simulink model "Charge_1_V1_experiment"  (R2018b)
settings: Solver=FixedStepDiscrete  StartTime=0.0  StopTime=1  FixedStep=0.001  RelTol=1e-3
PreLoadFcn:
  | librarySetup
  | eval([bdroot,'_startup']) %Calling [modelName]_startup.m
undefined symbols (not defined in the file or in its folder): A0, A1, Car1__Authorize, Car2_Authorize, CON2, CON3, CON4, Control_Mode_In, CurrentSP, D10, D12, D13, D2, D3, D4, D5, D6, D7, D8, Free_Charge, Frequency_High_Point, Frequency_Low_Point, Frequency_Mid_high, Frequency_Mid_low, HVol_High_Point, HVol_Low_Point, HVol_Mid_high, HVol_Mid_low, HVoltage_Factor, SeconCar_ThreePhase, V_Current_five, V_Current_four, V_Current_one, V_Current_six, V_Current_three, V_Current_two, V_Frequency, V_MaxPliot, V_MinPliot, Vol_High_Point, Vol_Low_Point, Vol_Mid_high, Vol_Mid_low, Voltage_Factor, Voltage_Mode_Test
libraries: simulink x324, HANcoder_STM32_Target x30, powerlib_meascontrol x8, simulink_extras x2
(part 10 of 13)

== system Charge_1_V1_experiment/HANcoder STM32 Target - E407-STM32 algorithm/Energy Meter/Energy_Meter_Recieve/Subsystem1/f1/Last byte ==
  note: 01040000000271CB
  Trigger : TriggerPort  VariantControl=Variant
  Constant1 : Constant  Value=hex2dec('0A')  OutDataTypeStr=uint8  SampleTime=-1
  UART send : Subsystem  Tag=HANcoder_TARGET_STM32_E407  AncestorBlock=HANcoder_STM32_Target/STM32-E407/UART/UART send  mask(UART send){channel=UART1: CON3 - D1 & D0, useStatusOut=off, tsamp=-1}
      mask prompts: useStatusOut "Use status outport"; tsamp "Sample time"
      mask help:
      | Function
      | ==========
      | Transmits a byte on the UART communication interface.
      |
      | Parameters per channel
      | ======================
      | - Select channel (TX & RX)
      | - Select if the status output should be enabled.
      |
      | Inputs
      | ======
      | - The byte to send
      |
      | Outputs
      | =======
      | - When the status output is 0, the byte could not be transmitted. Probably
      |   because the transmit buffer was configured too small.
      mask init:
      | uartChannelInfoStr = sfcn_uart_send_mcb(2, channel, useStatusOut);
      settings: MoveFcn=drawLogos
      mask Help: web('sfcn_uart_send.html')
      mask TypeOptions channel: UART1: CON3 - D1 & D0 | UART2: CON PD - 8 & 9 | UART3: CON PD - 11 & 12 | UART6: UEXT - 3 & 4
      mask Display: fprintf('UART send\n%s', uartChannelInfoStr);patch([245 251 251],[8 14 2],[1 0 0]);patch([253 253 259],[14 2 8],[0 0 0.35]);
  wires:
  Constant1/1 -> UART send/1(In1)

== system Charge_1_V1_experiment/HANcoder STM32 Target - E407-STM32 algorithm/Energy Meter/Energy_Meter_Recieve/Subsystem1/f1/Read_Gyro11 ==
  Trigger : TriggerPort  VariantControl=Variant
  Constant : Constant  Value=hex2dec('0E')  OutDataTypeStr=uint8  SampleTime=-1
  UART send : Subsystem  Tag=HANcoder_TARGET_STM32_E407  AncestorBlock=HANcoder_STM32_Target/STM32-E407/UART/UART send  mask(UART send){channel=UART1: CON3 - D1 & D0, useStatusOut=off, tsamp=-1}
      mask prompts: useStatusOut "Use status outport"; tsamp "Sample time"
      mask help:
      | Function
      | ==========
      | Transmits a byte on the UART communication interface.
      |
      | Parameters per channel
      | ======================
      | - Select channel (TX & RX)
      | - Select if the status output should be enabled.
      |
      | Inputs
      | ======
      | - The byte to send
      |
      | Outputs
      | =======
      | - When the status output is 0, the byte could not be transmitted. Probably
      |   because the transmit buffer was configured too small.
      mask init:
      | uartChannelInfoStr = sfcn_uart_send_mcb(2, channel, useStatusOut);
      settings: MoveFcn=drawLogos
      mask Help: web('sfcn_uart_send.html')
      mask TypeOptions channel: UART1: CON3 - D1 & D0 | UART2: CON PD - 8 & 9 | UART3: CON PD - 11 & 12 | UART6: UEXT - 3 & 4
      mask Display: fprintf('UART send\n%s', uartChannelInfoStr);patch([245 251 251],[8 14 2],[1 0 0]);patch([253 253 259],[14 2 8],[0 0 0.35]);
  wires:
  Constant/1 -> UART send/1(In1)

== system Charge_1_V1_experiment/HANcoder STM32 Target - E407-STM32 algorithm/Energy Meter/Energy_Meter_Recieve/Subsystem1/f1/Read_Gyro6 ==
  Trigger : TriggerPort  VariantControl=Variant
  Constant : Constant  Value=hex2dec('2')  OutDataTypeStr=uint8  SampleTime=-1
  UART send : Subsystem  Tag=HANcoder_TARGET_STM32_E407  AncestorBlock=HANcoder_STM32_Target/STM32-E407/UART/UART send  mask(UART send){channel=UART1: CON3 - D1 & D0, useStatusOut=off, tsamp=-1}
      mask prompts: useStatusOut "Use status outport"; tsamp "Sample time"
      mask help:
      | Function
      | ==========
      | Transmits a byte on the UART communication interface.
      |
      | Parameters per channel
      | ======================
      | - Select channel (TX & RX)
      | - Select if the status output should be enabled.
      |
      | Inputs
      | ======
      | - The byte to send
      |
      | Outputs
      | =======
      | - When the status output is 0, the byte could not be transmitted. Probably
      |   because the transmit buffer was configured too small.
      mask init:
      | uartChannelInfoStr = sfcn_uart_send_mcb(2, channel, useStatusOut);
      settings: MoveFcn=drawLogos
      mask Help: web('sfcn_uart_send.html')
      mask TypeOptions channel: UART1: CON3 - D1 & D0 | UART2: CON PD - 8 & 9 | UART3: CON PD - 11 & 12 | UART6: UEXT - 3 & 4
      mask Display: fprintf('UART send\n%s', uartChannelInfoStr);patch([245 251 251],[8 14 2],[1 0 0]);patch([253 253 259],[14 2 8],[0 0 0.35]);
  wires:
  Constant/1 -> UART send/1(In1)

== system Charge_1_V1_experiment/HANcoder STM32 Target - E407-STM32 algorithm/Energy Meter/Energy_Meter_Recieve/Subsystem1/f1/Subsystem ==
  In1 : Inport
  In10 : Inport  Port=2
  In11 : Inport  Port=3
  In12 : Inport  Port=4
  In13 : Inport  Port=5
  Compare To Constant10 : simulink/Logic and Bit Operations/Compare To Constant  relop===  const=411  OutDataTypeStr=boolean
  Compare To Constant11 : simulink/Logic and Bit Operations/Compare To Constant  relop===  const=412  OutDataTypeStr=boolean
  Compare To Constant13 : simulink/Logic and Bit Operations/Compare To Constant  relop===  const=413  OutDataTypeStr=boolean
  Compare To Constant9 : simulink/Logic and Bit Operations/Compare To Constant  relop===  const=410  OutDataTypeStr=boolean
  Read_Gyro10 : Subsystem  TreatAsAtomicUnit=on
  Read_Gyro12 : Subsystem  TreatAsAtomicUnit=on
  Read_Gyro13 : Subsystem  TreatAsAtomicUnit=on
  Read_Gyro14 : Subsystem  TreatAsAtomicUnit=on
  wires:
  In13/1 -> Read_Gyro14/1(In1)
  Compare To Constant13/1 -> Read_Gyro14/Trigger
  Compare To Constant11/1 -> Read_Gyro13/Trigger
  Compare To Constant9/1 -> Read_Gyro10/Trigger
  Compare To Constant10/1 -> Read_Gyro12/Trigger
  In12/1 -> Read_Gyro13/1(In1)
  In11/1 -> Read_Gyro12/1(In1)
  In10/1 -> Read_Gyro10/1(In1)
  In1/1 -> Compare To Constant9/1, Compare To Constant10/1, Compare To Constant11/1, Compare To Constant13/1

== system Charge_1_V1_experiment/HANcoder STM32 Target - E407-STM32 algorithm/Energy Meter/Energy_Meter_Recieve/Subsystem1/f2/Current_Phase1 ==
  In1 : Inport
  In2 : Inport  Port=2
  In3 : Inport  Port=3
  In4 : Inport  Port=4
  In5 : Inport  Port=5
  Compare To Constant1 : simulink/Logic and Bit Operations/Compare To Constant  relop===  const=603  OutDataTypeStr=boolean
  Compare To Constant12 : simulink/Logic and Bit Operations/Compare To Constant  relop===  const=602  OutDataTypeStr=boolean
  Compare To Constant2 : simulink/Logic and Bit Operations/Compare To Constant  relop===  const=604  OutDataTypeStr=boolean
  Compare To Constant3 : simulink/Logic and Bit Operations/Compare To Constant  relop===  const=605  OutDataTypeStr=boolean
  Read_Gyro1 : Subsystem  TreatAsAtomicUnit=on
  Read_Gyro2 : Subsystem  TreatAsAtomicUnit=on
  Read_Gyro3 : Subsystem  TreatAsAtomicUnit=on
  Read_Gyro4 : Subsystem  TreatAsAtomicUnit=on
  wires:
  In3/1 -> Read_Gyro2/1(In1)
  In2/1 -> Read_Gyro1/1(In1)
  Compare To Constant1/1 -> Read_Gyro2/Trigger
  Compare To Constant3/1 -> Read_Gyro4/Trigger
  Compare To Constant2/1 -> Read_Gyro3/Trigger
  In5/1 -> Read_Gyro4/1(In1)
  In4/1 -> Read_Gyro3/1(In1)
  Compare To Constant12/1 -> Read_Gyro1/Trigger
  In1/1 -> Compare To Constant3/1, Compare To Constant2/1, Compare To Constant1/1, Compare To Constant12/1

== system Charge_1_V1_experiment/HANcoder STM32 Target - E407-STM32 algorithm/Energy Meter/Energy_Meter_Recieve/Subsystem1/f2/Last byte ==
  note: 01040000000271CB
  Trigger : TriggerPort  VariantControl=Variant
  Constant1 : Constant  Value=hex2dec('0A')  OutDataTypeStr=uint8  SampleTime=-1
  UART send : Subsystem  Tag=HANcoder_TARGET_STM32_E407  AncestorBlock=HANcoder_STM32_Target/STM32-E407/UART/UART send  mask(UART send){channel=UART1: CON3 - D1 & D0, useStatusOut=off, tsamp=-1}
      mask prompts: useStatusOut "Use status outport"; tsamp "Sample time"
      mask help:
      | Function
      | ==========
      | Transmits a byte on the UART communication interface.
      |
      | Parameters per channel
      | ======================
      | - Select channel (TX & RX)
      | - Select if the status output should be enabled.
      |
      | Inputs
      | ======
      | - The byte to send
      |
      | Outputs
      | =======
      | - When the status output is 0, the byte could not be transmitted. Probably
      |   because the transmit buffer was configured too small.
      mask init:
      | uartChannelInfoStr = sfcn_uart_send_mcb(2, channel, useStatusOut);
      settings: MoveFcn=drawLogos
      mask Help: web('sfcn_uart_send.html')
      mask TypeOptions channel: UART1: CON3 - D1 & D0 | UART2: CON PD - 8 & 9 | UART3: CON PD - 11 & 12 | UART6: UEXT - 3 & 4
      mask Display: fprintf('UART send\n%s', uartChannelInfoStr);patch([245 251 251],[8 14 2],[1 0 0]);patch([253 253 259],[14 2 8],[0 0 0.35]);
  wires:
  Constant1/1 -> UART send/1(In1)

== system Charge_1_V1_experiment/HANcoder STM32 Target - E407-STM32 algorithm/Energy Meter/Energy_Meter_Recieve/Subsystem1/f2/Read_Gyro11 ==
  Trigger : TriggerPort  VariantControl=Variant
  Constant : Constant  Value=hex2dec('0F')  OutDataTypeStr=uint8  SampleTime=-1
  UART send : Subsystem  Tag=HANcoder_TARGET_STM32_E407  AncestorBlock=HANcoder_STM32_Target/STM32-E407/UART/UART send  mask(UART send){channel=UART1: CON3 - D1 & D0, useStatusOut=off, tsamp=-1}
      mask prompts: useStatusOut "Use status outport"; tsamp "Sample time"
      mask help:
      | Function
      | ==========
      | Transmits a byte on the UART communication interface.
      |
      | Parameters per channel
      | ======================
      | - Select channel (TX & RX)
      | - Select if the status output should be enabled.
      |
      | Inputs
      | ======
      | - The byte to send
      |
      | Outputs
      | =======
      | - When the status output is 0, the byte could not be transmitted. Probably
      |   because the transmit buffer was configured too small.
      mask init:
      | uartChannelInfoStr = sfcn_uart_send_mcb(2, channel, useStatusOut);
      settings: MoveFcn=drawLogos
      mask Help: web('sfcn_uart_send.html')
      mask TypeOptions channel: UART1: CON3 - D1 & D0 | UART2: CON PD - 8 & 9 | UART3: CON PD - 11 & 12 | UART6: UEXT - 3 & 4
      mask Display: fprintf('UART send\n%s', uartChannelInfoStr);patch([245 251 251],[8 14 2],[1 0 0]);patch([253 253 259],[14 2 8],[0 0 0.35]);
  wires:
  Constant/1 -> UART send/1(In1)

== system Charge_1_V1_experiment/HANcoder STM32 Target - E407-STM32 algorithm/Energy Meter/Energy_Meter_Recieve/Subsystem1/f2/Read_Gyro6 ==
  Trigger : TriggerPort  VariantControl=Variant
  Constant : Constant  Value=hex2dec('3')  OutDataTypeStr=uint8  SampleTime=-1
  UART send : Subsystem  Tag=HANcoder_TARGET_STM32_E407  AncestorBlock=HANcoder_STM32_Target/STM32-E407/UART/UART send  mask(UART send){channel=UART1: CON3 - D1 & D0, useStatusOut=off, tsamp=-1}
      mask prompts: useStatusOut "Use status outport"; tsamp "Sample time"
      mask help:
      | Function
      | ==========
      | Transmits a byte on the UART communication interface.
      |
      | Parameters per channel
      | ======================
      | - Select channel (TX & RX)
      | - Select if the status output should be enabled.
      |
      | Inputs
      | ======
      | - The byte to send
      |
      | Outputs
      | =======
      | - When the status output is 0, the byte could not be transmitted. Probably
      |   because the transmit buffer was configured too small.
      mask init:
      | uartChannelInfoStr = sfcn_uart_send_mcb(2, channel, useStatusOut);
      settings: MoveFcn=drawLogos
      mask Help: web('sfcn_uart_send.html')
      mask TypeOptions channel: UART1: CON3 - D1 & D0 | UART2: CON PD - 8 & 9 | UART3: CON PD - 11 & 12 | UART6: UEXT - 3 & 4
      mask Display: fprintf('UART send\n%s', uartChannelInfoStr);patch([245 251 251],[8 14 2],[1 0 0]);patch([253 253 259],[14 2 8],[0 0 0.35]);
  wires:
  Constant/1 -> UART send/1(In1)

== system Charge_1_V1_experiment/HANcoder STM32 Target - E407-STM32 algorithm/Energy Meter/Energy_Meter_Recieve/Voltage_meter1/Read_Gyro/UART receive ==
  Level-2 M-file S-Function : M-S-Function  Tag=XECU_TARGET_STM32_E407  FunctionName=sfcn_uart_receive  Parameters=tsamp
  Term1 : Terminator
  Out1 : Outport
  wires:
  Level-2 M-file S-Function/2 -> Term1/1
  Level-2 M-file S-Function/1 -> Out1/1

== system Charge_1_V1_experiment/HANcoder STM32 Target - E407-STM32 algorithm/Energy Meter/Energy_Meter_Recieve/Voltage_meter1/Read_Gyro1/UART receive ==
  Level-2 M-file S-Function : M-S-Function  Tag=XECU_TARGET_STM32_E407  FunctionName=sfcn_uart_receive  Parameters=tsamp
  Term1 : Terminator
  Out1 : Outport
  wires:
  Level-2 M-file S-Function/2 -> Term1/1
  Level-2 M-file S-Function/1 -> Out1/1

== system Charge_1_V1_experiment/HANcoder STM32 Target - E407-STM32 algorithm/Energy Meter/Energy_Meter_Recieve/Voltage_meter1/Read_Gyro10/UART receive ==
  Level-2 M-file S-Function : M-S-Function  Tag=XECU_TARGET_STM32_E407  FunctionName=sfcn_uart_receive  Parameters=tsamp
  Term1 : Terminator
  Out1 : Outport
  wires:
  Level-2 M-file S-Function/2 -> Term1/1
  Level-2 M-file S-Function/1 -> Out1/1

== system Charge_1_V1_experiment/HANcoder STM32 Target - E407-STM32 algorithm/Energy Meter/Energy_Meter_Recieve/Voltage_meter1/Read_Gyro11/UART receive ==
  Level-2 M-file S-Function : M-S-Function  Tag=XECU_TARGET_STM32_E407  FunctionName=sfcn_uart_receive  Parameters=tsamp
  Term1 : Terminator
  Out1 : Outport
  wires:
  Level-2 M-file S-Function/1 -> Out1/1
  Level-2 M-file S-Function/2 -> Term1/1

== system Charge_1_V1_experiment/HANcoder STM32 Target - E407-STM32 algorithm/Energy Meter/Energy_Meter_Recieve/Voltage_meter1/Read_Gyro12/UART receive ==
  Level-2 M-file S-Function : M-S-Function  Tag=XECU_TARGET_STM32_E407  FunctionName=sfcn_uart_receive  Parameters=tsamp
  Term1 : Terminator
  Out1 : Outport
  wires:
  Level-2 M-file S-Function/2 -> Term1/1
  Level-2 M-file S-Function/1 -> Out1/1

== system Charge_1_V1_experiment/HANcoder STM32 Target - E407-STM32 algorithm/Energy Meter/Energy_Meter_Recieve/Voltage_meter1/Read_Gyro13/UART receive ==
  Level-2 M-file S-Function : M-S-Function  Tag=XECU_TARGET_STM32_E407  FunctionName=sfcn_uart_receive  Parameters=tsamp
  Term1 : Terminator
  Out1 : Outport
  wires:
  Level-2 M-file S-Function/1 -> Out1/1
  Level-2 M-file S-Function/2 -> Term1/1

== system Charge_1_V1_experiment/HANcoder STM32 Target - E407-STM32 algorithm/Energy Meter/Energy_Meter_Recieve/Voltage_meter1/Read_Gyro14/UART receive ==
  Level-2 M-file S-Function : M-S-Function  Tag=XECU_TARGET_STM32_E407  FunctionName=sfcn_uart_receive  Parameters=tsamp
  Term1 : Terminator
  Out1 : Outport
  wires:
  Level-2 M-file S-Function/2 -> Term1/1
  Level-2 M-file S-Function/1 -> Out1/1

== system Charge_1_V1_experiment/HANcoder STM32 Target - E407-STM32 algorithm/Energy Meter/Energy_Meter_Recieve/Voltage_meter1/Read_Gyro15/UART receive ==
  Level-2 M-file S-Function : M-S-Function  Tag=XECU_TARGET_STM32_E407  FunctionName=sfcn_uart_receive  Parameters=tsamp
  Term1 : Terminator
  Out1 : Outport
  wires:
  Level-2 M-file S-Function/1 -> Out1/1
  Level-2 M-file S-Function/2 -> Term1/1

== system Charge_1_V1_experiment/HANcoder STM32 Target - E407-STM32 algorithm/Energy Meter/Energy_Meter_Recieve/Voltage_meter1/Read_Gyro16/UART receive ==
  Level-2 M-file S-Function : M-S-Function  Tag=XECU_TARGET_STM32_E407  FunctionName=sfcn_uart_receive  Parameters=tsamp
  Term1 : Terminator
  Out1 : Outport
  wires:
  Level-2 M-file S-Function/2 -> Term1/1
  Level-2 M-file S-Function/1 -> Out1/1

== system Charge_1_V1_experiment/HANcoder STM32 Target - E407-STM32 algorithm/Energy Meter/Energy_Meter_Recieve/Voltage_meter1/Read_Gyro17/UART receive ==
  Level-2 M-file S-Function : M-S-Function  Tag=XECU_TARGET_STM32_E407  FunctionName=sfcn_uart_receive  Parameters=tsamp
  Term1 : Terminator
  Out1 : Outport
  wires:
  Level-2 M-file S-Function/1 -> Out1/1
  Level-2 M-file S-Function/2 -> Term1/1

== system Charge_1_V1_experiment/HANcoder STM32 Target - E407-STM32 algorithm/Energy Meter/Energy_Meter_Recieve/Voltage_meter1/Read_Gyro2/UART receive ==
  Level-2 M-file S-Function : M-S-Function  Tag=XECU_TARGET_STM32_E407  FunctionName=sfcn_uart_receive  Parameters=tsamp
  Term1 : Terminator
  Out1 : Outport
  wires:
  Level-2 M-file S-Function/2 -> Term1/1
  Level-2 M-file S-Function/1 -> Out1/1

== system Charge_1_V1_experiment/HANcoder STM32 Target - E407-STM32 algorithm/Energy Meter/Energy_Meter_Recieve/Voltage_meter1/Read_Gyro3/UART receive ==
  Level-2 M-file S-Function : M-S-Function  Tag=XECU_TARGET_STM32_E407  FunctionName=sfcn_uart_receive  Parameters=tsamp
  Term1 : Terminator
  Out1 : Outport
  wires:
  Level-2 M-file S-Function/2 -> Term1/1
  Level-2 M-file S-Function/1 -> Out1/1

== system Charge_1_V1_experiment/HANcoder STM32 Target - E407-STM32 algorithm/Energy Meter/Energy_Meter_Recieve/Voltage_meter1/Read_Gyro4/UART receive ==
  Level-2 M-file S-Function : M-S-Function  Tag=XECU_TARGET_STM32_E407  FunctionName=sfcn_uart_receive  Parameters=tsamp
  Term1 : Terminator
  Out1 : Outport
  wires:
  Level-2 M-file S-Function/2 -> Term1/1
  Level-2 M-file S-Function/1 -> Out1/1

== system Charge_1_V1_experiment/HANcoder STM32 Target - E407-STM32 algorithm/Energy Meter/Energy_Meter_Recieve/Voltage_meter1/Read_Gyro5/UART receive ==
  Level-2 M-file S-Function : M-S-Function  Tag=XECU_TARGET_STM32_E407  FunctionName=sfcn_uart_receive  Parameters=tsamp
  Term1 : Terminator
  Out1 : Outport
  wires:
  Level-2 M-file S-Function/2 -> Term1/1
  Level-2 M-file S-Function/1 -> Out1/1

== system Charge_1_V1_experiment/HANcoder STM32 Target - E407-STM32 algorithm/Energy Meter/Energy_Meter_Recieve/Voltage_meter1/Read_Gyro6/UART receive ==
  Level-2 M-file S-Function : M-S-Function  Tag=XECU_TARGET_STM32_E407  FunctionName=sfcn_uart_receive  Parameters=tsamp
  Term1 : Terminator
  Out1 : Outport
  wires:
  Level-2 M-file S-Function/2 -> Term1/1
  Level-2 M-file S-Function/1 -> Out1/1

== system Charge_1_V1_experiment/HANcoder STM32 Target - E407-STM32 algorithm/Energy Meter/Energy_Meter_Recieve/Voltage_meter1/Read_Gyro7/UART receive ==
  Level-2 M-file S-Function : M-S-Function  Tag=XECU_TARGET_STM32_E407  FunctionName=sfcn_uart_receive  Parameters=tsamp
  Term1 : Terminator
  Out1 : Outport
  wires:
  Level-2 M-file S-Function/2 -> Term1/1
  Level-2 M-file S-Function/1 -> Out1/1

== system Charge_1_V1_experiment/HANcoder STM32 Target - E407-STM32 algorithm/Energy Meter/Energy_Meter_Recieve/Voltage_meter1/Read_Gyro8/UART receive ==
  Level-2 M-file S-Function : M-S-Function  Tag=XECU_TARGET_STM32_E407  FunctionName=sfcn_uart_receive  Parameters=tsamp
  Term1 : Terminator
  Out1 : Outport
  wires:
  Level-2 M-file S-Function/2 -> Term1/1
  Level-2 M-file S-Function/1 -> Out1/1

== system Charge_1_V1_experiment/HANcoder STM32 Target - E407-STM32 algorithm/Energy Meter/Energy_Meter_Recieve/Voltage_meter1/Read_Gyro9/UART receive ==
  Level-2 M-file S-Function : M-S-Function  Tag=XECU_TARGET_STM32_E407  FunctionName=sfcn_uart_receive  Parameters=tsamp
  Term1 : Terminator
  Out1 : Outport
  wires:
  Level-2 M-file S-Function/2 -> Term1/1
  Level-2 M-file S-Function/1 -> Out1/1

== system Charge_1_V1_experiment/HANcoder STM32 Target - E407-STM32 algorithm/Energy Meter/Energy_Meter_Recieve/Voltage_meter2/Read_Gyro/UART receive ==
  Level-2 M-file S-Function : M-S-Function  Tag=XECU_TARGET_STM32_E407  FunctionName=sfcn_uart_receive  Parameters=tsamp
  Term1 : Terminator
  Out1 : Outport
  wires:
  Level-2 M-file S-Function/1 -> Out1/1
  Level-2 M-file S-Function/2 -> Term1/1

== system Charge_1_V1_experiment/HANcoder STM32 Target - E407-STM32 algorithm/Energy Meter/Energy_Meter_Recieve/Voltage_meter2/Read_Gyro1/UART receive ==
  Level-2 M-file S-Function : M-S-Function  Tag=XECU_TARGET_STM32_E407  FunctionName=sfcn_uart_receive  Parameters=tsamp
  Term1 : Terminator
  Out1 : Outport
  wires:
  Level-2 M-file S-Function/1 -> Out1/1
  Level-2 M-file S-Function/2 -> Term1/1

== system Charge_1_V1_experiment/HANcoder STM32 Target - E407-STM32 algorithm/Energy Meter/Energy_Meter_Recieve/Voltage_meter2/Read_Gyro10/UART receive ==
  Level-2 M-file S-Function : M-S-Function  Tag=XECU_TARGET_STM32_E407  FunctionName=sfcn_uart_receive  Parameters=tsamp
  Term1 : Terminator
  Out1 : Outport
  wires:
  Level-2 M-file S-Function/1 -> Out1/1
  Level-2 M-file S-Function/2 -> Term1/1

== system Charge_1_V1_experiment/HANcoder STM32 Target - E407-STM32 algorithm/Energy Meter/Energy_Meter_Recieve/Voltage_meter2/Read_Gyro11/UART receive ==
  Level-2 M-file S-Function : M-S-Function  Tag=XECU_TARGET_STM32_E407  FunctionName=sfcn_uart_receive  Parameters=tsamp
  Term1 : Terminator
  Out1 : Outport
  wires:
  Level-2 M-file S-Function/2 -> Term1/1
  Level-2 M-file S-Function/1 -> Out1/1

== system Charge_1_V1_experiment/HANcoder STM32 Target - E407-STM32 algorithm/Energy Meter/Energy_Meter_Recieve/Voltage_meter2/Read_Gyro12/UART receive ==
  Level-2 M-file S-Function : M-S-Function  Tag=XECU_TARGET_STM32_E407  FunctionName=sfcn_uart_receive  Parameters=tsamp
  Term1 : Terminator
  Out1 : Outport
  wires:
  Level-2 M-file S-Function/1 -> Out1/1
  Level-2 M-file S-Function/2 -> Term1/1

== system Charge_1_V1_experiment/HANcoder STM32 Target - E407-STM32 algorithm/Energy Meter/Energy_Meter_Recieve/Voltage_meter2/Read_Gyro13/UART receive ==
  Level-2 M-file S-Function : M-S-Function  Tag=XECU_TARGET_STM32_E407  FunctionName=sfcn_uart_receive  Parameters=tsamp
  Term1 : Terminator
  Out1 : Outport
  wires:
  Level-2 M-file S-Function/2 -> Term1/1
  Level-2 M-file S-Function/1 -> Out1/1

== system Charge_1_V1_experiment/HANcoder STM32 Target - E407-STM32 algorithm/Energy Meter/Energy_Meter_Recieve/Voltage_meter2/Read_Gyro14/UART receive ==
  Level-2 M-file S-Function : M-S-Function  Tag=XECU_TARGET_STM32_E407  FunctionName=sfcn_uart_receive  Parameters=tsamp
  Term1 : Terminator
  Out1 : Outport
  wires:
  Level-2 M-file S-Function/1 -> Out1/1
  Level-2 M-file S-Function/2 -> Term1/1

== system Charge_1_V1_experiment/HANcoder STM32 Target - E407-STM32 algorithm/Energy Meter/Energy_Meter_Recieve/Voltage_meter2/Read_Gyro15/UART receive ==
  Level-2 M-file S-Function : M-S-Function  Tag=XECU_TARGET_STM32_E407  FunctionName=sfcn_uart_receive  Parameters=tsamp
  Term1 : Terminator
  Out1 : Outport
  wires:
  Level-2 M-file S-Function/2 -> Term1/1
  Level-2 M-file S-Function/1 -> Out1/1

== system Charge_1_V1_experiment/HANcoder STM32 Target - E407-STM32 algorithm/Energy Meter/Energy_Meter_Recieve/Voltage_meter2/Read_Gyro16/UART receive ==
  Level-2 M-file S-Function : M-S-Function  Tag=XECU_TARGET_STM32_E407  FunctionName=sfcn_uart_receive  Parameters=tsamp
  Term1 : Terminator
  Out1 : Outport
  wires:
  Level-2 M-file S-Function/1 -> Out1/1
  Level-2 M-file S-Function/2 -> Term1/1

== system Charge_1_V1_experiment/HANcoder STM32 Target - E407-STM32 algorithm/Energy Meter/Energy_Meter_Recieve/Voltage_meter2/Read_Gyro17/UART receive ==
  Level-2 M-file S-Function : M-S-Function  Tag=XECU_TARGET_STM32_E407  FunctionName=sfcn_uart_receive  Parameters=tsamp
  Term1 : Terminator
  Out1 : Outport
  wires:
  Level-2 M-file S-Function/2 -> Term1/1
  Level-2 M-file S-Function/1 -> Out1/1

== system Charge_1_V1_experiment/HANcoder STM32 Target - E407-STM32 algorithm/Energy Meter/Energy_Meter_Recieve/Voltage_meter2/Read_Gyro2/UART receive ==
  Level-2 M-file S-Function : M-S-Function  Tag=XECU_TARGET_STM32_E407  FunctionName=sfcn_uart_receive  Parameters=tsamp
  Term1 : Terminator
  Out1 : Outport
  wires:
  Level-2 M-file S-Function/1 -> Out1/1
  Level-2 M-file S-Function/2 -> Term1/1

== system Charge_1_V1_experiment/HANcoder STM32 Target - E407-STM32 algorithm/Energy Meter/Energy_Meter_Recieve/Voltage_meter2/Read_Gyro3/UART receive ==
  Level-2 M-file S-Function : M-S-Function  Tag=XECU_TARGET_STM32_E407  FunctionName=sfcn_uart_receive  Parameters=tsamp
  Term1 : Terminator
  Out1 : Outport
  wires:
  Level-2 M-file S-Function/1 -> Out1/1
  Level-2 M-file S-Function/2 -> Term1/1

== system Charge_1_V1_experiment/HANcoder STM32 Target - E407-STM32 algorithm/Energy Meter/Energy_Meter_Recieve/Voltage_meter2/Read_Gyro4/UART receive ==
  Level-2 M-file S-Function : M-S-Function  Tag=XECU_TARGET_STM32_E407  FunctionName=sfcn_uart_receive  Parameters=tsamp
  Term1 : Terminator
  Out1 : Outport
  wires:
  Level-2 M-file S-Function/1 -> Out1/1
  Level-2 M-file S-Function/2 -> Term1/1

== system Charge_1_V1_experiment/HANcoder STM32 Target - E407-STM32 algorithm/Energy Meter/Energy_Meter_Recieve/Voltage_meter2/Read_Gyro5/UART receive ==
  Level-2 M-file S-Function : M-S-Function  Tag=XECU_TARGET_STM32_E407  FunctionName=sfcn_uart_receive  Parameters=tsamp
  Term1 : Terminator
  Out1 : Outport
  wires:
  Level-2 M-file S-Function/1 -> Out1/1
  Level-2 M-file S-Function/2 -> Term1/1

== system Charge_1_V1_experiment/HANcoder STM32 Target - E407-STM32 algorithm/Energy Meter/Energy_Meter_Recieve/Voltage_meter2/Read_Gyro6/UART receive ==
  Level-2 M-file S-Function : M-S-Function  Tag=XECU_TARGET_STM32_E407  FunctionName=sfcn_uart_receive  Parameters=tsamp
  Term1 : Terminator
  Out1 : Outport
  wires:
  Level-2 M-file S-Function/1 -> Out1/1
  Level-2 M-file S-Function/2 -> Term1/1

== system Charge_1_V1_experiment/HANcoder STM32 Target - E407-STM32 algorithm/Energy Meter/Energy_Meter_Recieve/Voltage_meter2/Read_Gyro7/UART receive ==
  Level-2 M-file S-Function : M-S-Function  Tag=XECU_TARGET_STM32_E407  FunctionName=sfcn_uart_receive  Parameters=tsamp
  Term1 : Terminator
  Out1 : Outport
  wires:
  Level-2 M-file S-Function/1 -> Out1/1
  Level-2 M-file S-Function/2 -> Term1/1

== system Charge_1_V1_experiment/HANcoder STM32 Target - E407-STM32 algorithm/Energy Meter/Energy_Meter_Recieve/Voltage_meter2/Read_Gyro8/UART receive ==
  Level-2 M-file S-Function : M-S-Function  Tag=XECU_TARGET_STM32_E407  FunctionName=sfcn_uart_receive  Parameters=tsamp
  Term1 : Terminator
  Out1 : Outport
  wires:
  Level-2 M-file S-Function/1 -> Out1/1
  Level-2 M-file S-Function/2 -> Term1/1

== system Charge_1_V1_experiment/HANcoder STM32 Target - E407-STM32 algorithm/Energy Meter/Energy_Meter_Recieve/Voltage_meter2/Read_Gyro9/UART receive ==
  Level-2 M-file S-Function : M-S-Function  Tag=XECU_TARGET_STM32_E407  FunctionName=sfcn_uart_receive  Parameters=tsamp
  Term1 : Terminator
  Out1 : Outport
  wires:
  Level-2 M-file S-Function/1 -> Out1/1
  Level-2 M-file S-Function/2 -> Term1/1

== system Charge_1_V1_experiment/HANcoder STM32 Target - E407-STM32 algorithm/Energy Meter/Energymeter_Request/Current_Meter_1 /Read_Gyro1/UART send ==
  In1 : Inport
  Level-2 M-file S-Function : M-S-Function  FunctionName=sfcn_uart_send  Parameters=tsamp
  Term1 : Terminator
  wires:
  In1/1 -> Level-2 M-file S-Function/1
  Level-2 M-file S-Function/1 -> Term1/1

== system Charge_1_V1_experiment/HANcoder STM32 Target - E407-STM32 algorithm/Energy Meter/Energymeter_Request/Current_Meter_1 /Read_Gyro2/UART send ==
  In1 : Inport
  Level-2 M-file S-Function : M-S-Function  FunctionName=sfcn_uart_send  Parameters=tsamp
  Term1 : Terminator
  wires:
  In1/1 -> Level-2 M-file S-Function/1
  Level-2 M-file S-Function/1 -> Term1/1

== system Charge_1_V1_experiment/HANcoder STM32 Target - E407-STM32 algorithm/Energy Meter/Energymeter_Request/Current_Meter_1 /Read_Gyro3/UART send ==
  In1 : Inport
  Level-2 M-file S-Function : M-S-Function  FunctionName=sfcn_uart_send  Parameters=tsamp
  Term1 : Terminator
  wires:
  In1/1 -> Level-2 M-file S-Function/1
  Level-2 M-file S-Function/1 -> Term1/1

== system Charge_1_V1_experiment/HANcoder STM32 Target - E407-STM32 algorithm/Energy Meter/Energymeter_Request/Current_Meter_1 /Read_Gyro4/UART send ==
  In1 : Inport
  Level-2 M-file S-Function : M-S-Function  FunctionName=sfcn_uart_send  Parameters=tsamp
  Term1 : Terminator
  wires:
  In1/1 -> Level-2 M-file S-Function/1
  Level-2 M-file S-Function/1 -> Term1/1

== system Charge_1_V1_experiment/HANcoder STM32 Target - E407-STM32 algorithm/Energy Meter/Energymeter_Request/Current_Meter_1 /Read_Gyro5/UART send ==
  In1 : Inport
  Level-2 M-file S-Function : M-S-Function  FunctionName=sfcn_uart_send  Parameters=tsamp
  Term1 : Terminator
  wires:
  In1/1 -> Level-2 M-file S-Function/1
  Level-2 M-file S-Function/1 -> Term1/1

== system Charge_1_V1_experiment/HANcoder STM32 Target - E407-STM32 algorithm/Energy Meter/Energymeter_Request/Current_Meter_1 /Read_Gyro6/UART send ==
  In1 : Inport
  Level-2 M-file S-Function : M-S-Function  FunctionName=sfcn_uart_send  Parameters=tsamp
  Term1 : Terminator
  wires:
  In1/1 -> Level-2 M-file S-Function/1
  Level-2 M-file S-Function/1 -> Term1/1

== system Charge_1_V1_experiment/HANcoder STM32 Target - E407-STM32 algorithm/Energy Meter/Energymeter_Request/Current_Meter_1 /Read_Gyro7/UART send ==
  In1 : Inport
  Level-2 M-file S-Function : M-S-Function  FunctionName=sfcn_uart_send  Parameters=tsamp
  Term1 : Terminator
  wires:
  In1/1 -> Level-2 M-file S-Function/1
  Level-2 M-file S-Function/1 -> Term1/1

== system Charge_1_V1_experiment/HANcoder STM32 Target - E407-STM32 algorithm/Energy Meter/Energymeter_Request/Current_Meter_1 /Read_Gyro8/UART send ==
  In1 : Inport
  Level-2 M-file S-Function : M-S-Function  FunctionName=sfcn_uart_send  Parameters=tsamp
  Term1 : Terminator
  wires:
  In1/1 -> Level-2 M-file S-Function/1
  Level-2 M-file S-Function/1 -> Term1/1

== system Charge_1_V1_experiment/HANcoder STM32 Target - E407-STM32 algorithm/Energy Meter/Energymeter_Request/Current_Meter_2/Read_Gyro10/UART send ==
  In1 : Inport
  Level-2 M-file S-Function : M-S-Function  FunctionName=sfcn_uart_send  Parameters=tsamp
  Term1 : Terminator
  wires:
  In1/1 -> Level-2 M-file S-Function/1
  Level-2 M-file S-Function/1 -> Term1/1

== system Charge_1_V1_experiment/HANcoder STM32 Target - E407-STM32 algorithm/Energy Meter/Energymeter_Request/Current_Meter_2/Read_Gyro11/UART send ==
  In1 : Inport
  Level-2 M-file S-Function : M-S-Function  FunctionName=sfcn_uart_send  Parameters=tsamp
  Term1 : Terminator
  wires:
  In1/1 -> Level-2 M-file S-Function/1
  Level-2 M-file S-Function/1 -> Term1/1

== system Charge_1_V1_experiment/HANcoder STM32 Target - E407-STM32 algorithm/Energy Meter/Energymeter_Request/Current_Meter_2/Read_Gyro12/UART send ==
  In1 : Inport
  Level-2 M-file S-Function : M-S-Function  FunctionName=sfcn_uart_send  Parameters=tsamp
  Term1 : Terminator
  wires:
  In1/1 -> Level-2 M-file S-Function/1
  Level-2 M-file S-Function/1 -> Term1/1

== system Charge_1_V1_experiment/HANcoder STM32 Target - E407-STM32 algorithm/Energy Meter/Energymeter_Request/Current_Meter_2/Read_Gyro13/UART send ==
  In1 : Inport
  Level-2 M-file S-Function : M-S-Function  FunctionName=sfcn_uart_send  Parameters=tsamp
  Term1 : Terminator
  wires:
  In1/1 -> Level-2 M-file S-Function/1
  Level-2 M-file S-Function/1 -> Term1/1

== system Charge_1_V1_experiment/HANcoder STM32 Target - E407-STM32 algorithm/Energy Meter/Energymeter_Request/Current_Meter_2/Read_Gyro14/UART send ==
  In1 : Inport
  Level-2 M-file S-Function : M-S-Function  FunctionName=sfcn_uart_send  Parameters=tsamp
  Term1 : Terminator
  wires:
  In1/1 -> Level-2 M-file S-Function/1
  Level-2 M-file S-Function/1 -> Term1/1

== system Charge_1_V1_experiment/HANcoder STM32 Target - E407-STM32 algorithm/Energy Meter/Energymeter_Request/Current_Meter_2/Read_Gyro15/UART send ==
  In1 : Inport
  Level-2 M-file S-Function : M-S-Function  FunctionName=sfcn_uart_send  Parameters=tsamp
  Term1 : Terminator
  wires:
  In1/1 -> Level-2 M-file S-Function/1
  Level-2 M-file S-Function/1 -> Term1/1

== system Charge_1_V1_experiment/HANcoder STM32 Target - E407-STM32 algorithm/Energy Meter/Energymeter_Request/Current_Meter_2/Read_Gyro16/UART send ==
  In1 : Inport
  Level-2 M-file S-Function : M-S-Function  FunctionName=sfcn_uart_send  Parameters=tsamp
  Term1 : Terminator
  wires:
  In1/1 -> Level-2 M-file S-Function/1
  Level-2 M-file S-Function/1 -> Term1/1

== system Charge_1_V1_experiment/HANcoder STM32 Target - E407-STM32 algorithm/Energy Meter/Energymeter_Request/Current_Meter_2/Read_Gyro9/UART send ==
  In1 : Inport
  Level-2 M-file S-Function : M-S-Function  FunctionName=sfcn_uart_send  Parameters=tsamp
  Term1 : Terminator
  wires:
  In1/1 -> Level-2 M-file S-Function/1
  Level-2 M-file S-Function/1 -> Term1/1

== system Charge_1_V1_experiment/HANcoder STM32 Target - E407-STM32 algorithm/Energy Meter/Energymeter_Request/Fequency/Read_Gyro10/UART send ==
  In1 : Inport
  Level-2 M-file S-Function : M-S-Function  FunctionName=sfcn_uart_send  Parameters=tsamp
  Term1 : Terminator
  wires:
  In1/1 -> Level-2 M-file S-Function/1
  Level-2 M-file S-Function/1 -> Term1/1

== system Charge_1_V1_experiment/HANcoder STM32 Target - E407-STM32 algorithm/Energy Meter/Energymeter_Request/Fequency/Read_Gyro11/UART send ==
  In1 : Inport
  Level-2 M-file S-Function : M-S-Function  FunctionName=sfcn_uart_send  Parameters=tsamp
  Term1 : Terminator
  wires:
  In1/1 -> Level-2 M-file S-Function/1
  Level-2 M-file S-Function/1 -> Term1/1

== system Charge_1_V1_experiment/HANcoder STM32 Target - E407-STM32 algorithm/Energy Meter/Energymeter_Request/Fequency/Read_Gyro12/UART send ==
  In1 : Inport
  Level-2 M-file S-Function : M-S-Function  FunctionName=sfcn_uart_send  Parameters=tsamp
  Term1 : Terminator
  wires:
  In1/1 -> Level-2 M-file S-Function/1
  Level-2 M-file S-Function/1 -> Term1/1

== system Charge_1_V1_experiment/HANcoder STM32 Target - E407-STM32 algorithm/Energy Meter/Energymeter_Request/Fequency/Read_Gyro13/UART send ==
  In1 : Inport
  Level-2 M-file S-Function : M-S-Function  FunctionName=sfcn_uart_send  Parameters=tsamp
  Term1 : Terminator
  wires:
  In1/1 -> Level-2 M-file S-Function/1
  Level-2 M-file S-Function/1 -> Term1/1

== system Charge_1_V1_experiment/HANcoder STM32 Target - E407-STM32 algorithm/Energy Meter/Energymeter_Request/Fequency/Read_Gyro14/UART send ==
  In1 : Inport
  Level-2 M-file S-Function : M-S-Function  FunctionName=sfcn_uart_send  Parameters=tsamp
  Term1 : Terminator
  wires:
  In1/1 -> Level-2 M-file S-Function/1
  Level-2 M-file S-Function/1 -> Term1/1

== system Charge_1_V1_experiment/HANcoder STM32 Target - E407-STM32 algorithm/Energy Meter/Energymeter_Request/Fequency/Read_Gyro15/UART send ==
  In1 : Inport
  Level-2 M-file S-Function : M-S-Function  FunctionName=sfcn_uart_send  Parameters=tsamp
  Term1 : Terminator
  wires:
  In1/1 -> Level-2 M-file S-Function/1
  Level-2 M-file S-Function/1 -> Term1/1

== system Charge_1_V1_experiment/HANcoder STM32 Target - E407-STM32 algorithm/Energy Meter/Energymeter_Request/Fequency/Read_Gyro16/UART send ==
  In1 : Inport
  Level-2 M-file S-Function : M-S-Function  FunctionName=sfcn_uart_send  Parameters=tsamp
  Term1 : Terminator
  wires:
  In1/1 -> Level-2 M-file S-Function/1
  Level-2 M-file S-Function/1 -> Term1/1

== system Charge_1_V1_experiment/HANcoder STM32 Target - E407-STM32 algorithm/Energy Meter/Energymeter_Request/Fequency/Read_Gyro9/UART send ==
  In1 : Inport
  Level-2 M-file S-Function : M-S-Function  FunctionName=sfcn_uart_send  Parameters=tsamp
  Term1 : Terminator
  wires:
  In1/1 -> Level-2 M-file S-Function/1
  Level-2 M-file S-Function/1 -> Term1/1

== system Charge_1_V1_experiment/HANcoder STM32 Target - E407-STM32 algorithm/Energy Meter/Energymeter_Request/Voltage_meter_1/Read_Gyro1/UART send ==
  In1 : Inport
  Level-2 M-file S-Function : M-S-Function  FunctionName=sfcn_uart_send  Parameters=tsamp
  Term1 : Terminator
  wires:
  Level-2 M-file S-Function/1 -> Term1/1
  In1/1 -> Level-2 M-file S-Function/1

== system Charge_1_V1_experiment/HANcoder STM32 Target - E407-STM32 algorithm/Energy Meter/Energymeter_Request/Voltage_meter_1/Read_Gyro2/UART send ==
  In1 : Inport
  Level-2 M-file S-Function : M-S-Function  FunctionName=sfcn_uart_send  Parameters=tsamp
  Term1 : Terminator
  wires:
  Level-2 M-file S-Function/1 -> Term1/1
  In1/1 -> Level-2 M-file S-Function/1

== system Charge_1_V1_experiment/HANcoder STM32 Target - E407-STM32 algorithm/Energy Meter/Energymeter_Request/Voltage_meter_1/Read_Gyro3/UART send ==
  In1 : Inport
  Level-2 M-file S-Function : M-S-Function  FunctionName=sfcn_uart_send  Parameters=tsamp
  Term1 : Terminator
  wires:
  Level-2 M-file S-Function/1 -> Term1/1
  In1/1 -> Level-2 M-file S-Function/1

== system Charge_1_V1_experiment/HANcoder STM32 Target - E407-STM32 algorithm/Energy Meter/Energymeter_Request/Voltage_meter_1/Read_Gyro4/UART send ==
  In1 : Inport
  Level-2 M-file S-Function : M-S-Function  FunctionName=sfcn_uart_send  Parameters=tsamp
  Term1 : Terminator
  wires:
  Level-2 M-file S-Function/1 -> Term1/1
  In1/1 -> Level-2 M-file S-Function/1

== system Charge_1_V1_experiment/HANcoder STM32 Target - E407-STM32 algorithm/Energy Meter/Energymeter_Request/Voltage_meter_1/Read_Gyro5/UART send ==
  In1 : Inport
  Level-2 M-file S-Function : M-S-Function  FunctionName=sfcn_uart_send  Parameters=tsamp
  Term1 : Terminator
  wires:
  Level-2 M-file S-Function/1 -> Term1/1
  In1/1 -> Level-2 M-file S-Function/1

== system Charge_1_V1_experiment/HANcoder STM32 Target - E407-STM32 algorithm/Energy Meter/Energymeter_Request/Voltage_meter_1/Read_Gyro6/UART send ==
  In1 : Inport
  Level-2 M-file S-Function : M-S-Function  FunctionName=sfcn_uart_send  Parameters=tsamp
  Term1 : Terminator
  wires:
  Level-2 M-file S-Function/1 -> Term1/1
  In1/1 -> Level-2 M-file S-Function/1

== system Charge_1_V1_experiment/HANcoder STM32 Target - E407-STM32 algorithm/Energy Meter/Energymeter_Request/Voltage_meter_1/Read_Gyro7/UART send ==
  In1 : Inport
  Level-2 M-file S-Function : M-S-Function  FunctionName=sfcn_uart_send  Parameters=tsamp
  Term1 : Terminator
  wires:
  Level-2 M-file S-Function/1 -> Term1/1
  In1/1 -> Level-2 M-file S-Function/1

== system Charge_1_V1_experiment/HANcoder STM32 Target - E407-STM32 algorithm/Energy Meter/Energymeter_Request/Voltage_meter_1/Read_Gyro8/UART send ==
  In1 : Inport
  Level-2 M-file S-Function : M-S-Function  FunctionName=sfcn_uart_send  Parameters=tsamp
  Term1 : Terminator
  wires:
  Level-2 M-file S-Function/1 -> Term1/1
  In1/1 -> Level-2 M-file S-Function/1

== system Charge_1_V1_experiment/HANcoder STM32 Target - E407-STM32 algorithm/Energy Meter/Energymeter_Request/Voltage_meter_2/Read_Gyro1/UART send ==
  In1 : Inport
  Level-2 M-file S-Function : M-S-Function  FunctionName=sfcn_uart_send  Parameters=tsamp
  Term1 : Terminator
  wires:
  In1/1 -> Level-2 M-file S-Function/1
  Level-2 M-file S-Function/1 -> Term1/1

== system Charge_1_V1_experiment/HANcoder STM32 Target - E407-STM32 algorithm/Energy Meter/Energymeter_Request/Voltage_meter_2/Read_Gyro2/UART send ==
  In1 : Inport
  Level-2 M-file S-Function : M-S-Function  FunctionName=sfcn_uart_send  Parameters=tsamp
  Term1 : Terminator
  wires:
  In1/1 -> Level-2 M-file S-Function/1
  Level-2 M-file S-Function/1 -> Term1/1

== system Charge_1_V1_experiment/HANcoder STM32 Target - E407-STM32 algorithm/Energy Meter/Energymeter_Request/Voltage_meter_2/Read_Gyro3/UART send ==
  In1 : Inport
  Level-2 M-file S-Function : M-S-Function  FunctionName=sfcn_uart_send  Parameters=tsamp
  Term1 : Terminator
  wires:
  In1/1 -> Level-2 M-file S-Function/1
  Level-2 M-file S-Function/1 -> Term1/1

== system Charge_1_V1_experiment/HANcoder STM32 Target - E407-STM32 algorithm/Energy Meter/Energymeter_Request/Voltage_meter_2/Read_Gyro4/UART send ==
  In1 : Inport
  Level-2 M-file S-Function : M-S-Function  FunctionName=sfcn_uart_send  Parameters=tsamp
  Term1 : Terminator
  wires:
  In1/1 -> Level-2 M-file S-Function/1
  Level-2 M-file S-Function/1 -> Term1/1

== system Charge_1_V1_experiment/HANcoder STM32 Target - E407-STM32 algorithm/Energy Meter/Energymeter_Request/Voltage_meter_2/Read_Gyro5/UART send ==
  In1 : Inport
  Level-2 M-file S-Function : M-S-Function  FunctionName=sfcn_uart_send  Parameters=tsamp
  Term1 : Terminator
  wires:
  In1/1 -> Level-2 M-file S-Function/1
  Level-2 M-file S-Function/1 -> Term1/1

== system Charge_1_V1_experiment/HANcoder STM32 Target - E407-STM32 algorithm/Energy Meter/Energymeter_Request/Voltage_meter_2/Read_Gyro6/UART send ==
  In1 : Inport
  Level-2 M-file S-Function : M-S-Function  FunctionName=sfcn_uart_send  Parameters=tsamp
  Term1 : Terminator
  wires:
  In1/1 -> Level-2 M-file S-Function/1
  Level-2 M-file S-Function/1 -> Term1/1

== system Charge_1_V1_experiment/HANcoder STM32 Target - E407-STM32 algorithm/Energy Meter/Energymeter_Request/Voltage_meter_2/Read_Gyro7/UART send ==
  In1 : Inport
  Level-2 M-file S-Function : M-S-Function  FunctionName=sfcn_uart_send  Parameters=tsamp
  Term1 : Terminator
  wires:
  In1/1 -> Level-2 M-file S-Function/1
  Level-2 M-file S-Function/1 -> Term1/1

== system Charge_1_V1_experiment/HANcoder STM32 Target - E407-STM32 algorithm/Energy Meter/Energymeter_Request/Voltage_meter_2/Read_Gyro8/UART send ==
  In1 : Inport
  Level-2 M-file S-Function : M-S-Function  FunctionName=sfcn_uart_send  Parameters=tsamp
  Term1 : Terminator
  wires:
  In1/1 -> Level-2 M-file S-Function/1
  Level-2 M-file S-Function/1 -> Term1/1

== system Charge_1_V1_experiment/HANcoder STM32 Target - E407-STM32 algorithm/Current_SP/Subsystem1/Voltage_Control/1phase/Subsystem/Subsystem ==
  In1 : Inport
  In2 : Inport  Port=2
  In3 : Inport  Port=3
  In4 : Inport  Port=4
  In5 : Inport  Port=5
  In6 : Inport  Port=6
  In7 : Inport  Port=7
  In8 : Inport  Port=8
  Constant10 : Constant  Value=5  OutDataTypeStr=single  SampleTime=-1
  Constant6 : Constant  OutDataTypeStr=single  SampleTime=-1
  Constant7 : Constant  Value=2  OutDataTypeStr=single  SampleTime=-1
  Constant8 : Constant  Value=3  OutDataTypeStr=single  SampleTime=-1
  Constant9 : Constant  Value=4  OutDataTypeStr=single  SampleTime=-1
  Logical Operator : Logic  AllPortsSameDT=off  OutDataTypeStr=boolean
  Logical Operator1 : Logic  AllPortsSameDT=off  OutDataTypeStr=boolean
  Logical Operator2 : Logic  AllPortsSameDT=off  OutDataTypeStr=boolean
  Switch{,1..4} (5 alike) : Switch  Criteria=u2 > Threshold
  Out1 : Outport
  wires:
  Logical Operator2/1 -> Switch3/2
  Switch3/1 -> Switch4/3
  Switch2/1 -> Switch3/3
  Constant8/1 -> Switch2/1
  Constant10/1 -> Switch4/1
  Constant7/1 -> Switch1/1
  Switch/1 -> Switch1/3
  Logical Operator/1 -> Switch1/2
  In8/1 -> Switch4/2
  Switch4/1 -> Out1/1
  Constant9/1 -> Switch3/1
  Switch1/1 -> Switch2/3
  In1/1 -> Switch/2
  Logical Operator1/1 -> Switch2/2
  In4/1 -> Logical Operator1/1
  In2/1 -> Logical Operator/1
  In5/1 -> Logical Operator1/2
  In3/1 -> Logical Operator/2
  In6/1 -> Logical Operator2/1
  In7/1 -> Logical Operator2/2
  Constant6/1 -> Switch/3, Switch/1

== system Charge_1_V1_experiment/HANcoder STM32 Target - E407-STM32 algorithm/Current_SP/Subsystem1/Voltage_Control/3phase/Subsystem1/Subsystem ==
  In1 : Inport
  In2 : Inport  Port=2
  In3 : Inport  Port=3
  In4 : Inport  Port=4
  In5 : Inport  Port=5
  In6 : Inport  Port=6
  In7 : Inport  Port=7
  In8 : Inport  Port=8
  Constant10 : Constant  Value=5  OutDataTypeStr=single  SampleTime=-1
  Constant6 : Constant  OutDataTypeStr=single  SampleTime=-1
  Constant7 : Constant  Value=2  OutDataTypeStr=single  SampleTime=-1
  Constant8 : Constant  Value=3  OutDataTypeStr=single  SampleTime=-1
  Constant9 : Constant  Value=4  OutDataTypeStr=single  SampleTime=-1
  Logical Operator : Logic  AllPortsSameDT=off  OutDataTypeStr=boolean
  Logical Operator1 : Logic  AllPortsSameDT=off  OutDataTypeStr=boolean
  Logical Operator2 : Logic  AllPortsSameDT=off  OutDataTypeStr=boolean
  Switch{,1..4} (5 alike) : Switch  Criteria=u2 > Threshold
  Out1 : Outport
  wires:
  Constant6/1 -> Switch/1, Switch/3
  In7/1 -> Logical Operator2/2
  In6/1 -> Logical Operator2/1
  In3/1 -> Logical Operator/2
  In5/1 -> Logical Operator1/2
  In2/1 -> Logical Operator/1
  In4/1 -> Logical Operator1/1
  Logical Operator1/1 -> Switch2/2
  In1/1 -> Switch/2
  Switch1/1 -> Switch2/3
  Constant9/1 -> Switch3/1
  Switch4/1 -> Out1/1
  In8/1 -> Switch4/2
  Logical Operator/1 -> Switch1/2
  Switch/1 -> Switch1/3
  Constant7/1 -> Switch1/1
  Constant10/1 -> Switch4/1
  Constant8/1 -> Switch2/1
  Switch2/1 -> Switch3/3
  Switch3/1 -> Switch4/3
  Logical Operator2/1 -> Switch3/2

== system Charge_1_V1_experiment/HANcoder STM32 Target - E407-STM32 algorithm/Current_SP/Subsystem2/Voltage_Control/1phase/Subsystem/Subsystem ==
  In1 : Inport
  In2 : Inport  Port=2
  In3 : Inport  Port=3
  In4 : Inport  Port=4
  In5 : Inport  Port=5
  In6 : Inport  Port=6
  In7 : Inport  Port=7
  In8 : Inport  Port=8
  Constant10 : Constant  Value=5  OutDataTypeStr=single  SampleTime=-1
  Constant6 : Constant  OutDataTypeStr=single  SampleTime=-1
  Constant7 : Constant  Value=2  OutDataTypeStr=single  SampleTime=-1
  Constant8 : Constant  Value=3  OutDataTypeStr=single  SampleTime=-1
  Constant9 : Constant  Value=4  OutDataTypeStr=single  SampleTime=-1
  Logical Operator : Logic  AllPortsSameDT=off  OutDataTypeStr=boolean
  Logical Operator1 : Logic  AllPortsSameDT=off  OutDataTypeStr=boolean
  Logical Operator2 : Logic  AllPortsSameDT=off  OutDataTypeStr=boolean
  Switch{,1..4} (5 alike) : Switch  Criteria=u2 > Threshold
  Out1 : Outport
  wires:
  Logical Operator2/1 -> Switch3/2
  Switch3/1 -> Switch4/3
  Switch2/1 -> Switch3/3
  Constant8/1 -> Switch2/1
  Constant10/1 -> Switch4/1
  Constant7/1 -> Switch1/1
  Switch/1 -> Switch1/3
  Logical Operator/1 -> Switch1/2
  In8/1 -> Switch4/2
  Switch4/1 -> Out1/1
  Constant9/1 -> Switch3/1
  Switch1/1 -> Switch2/3
  In1/1 -> Switch/2
  Logical Operator1/1 -> Switch2/2
  In4/1 -> Logical Operator1/1
  In2/1 -> Logical Operator/1
  In5/1 -> Logical Operator1/2
  In3/1 -> Logical Operator/2
  In6/1 -> Logical Operator2/1
  In7/1 -> Logical Operator2/2
  Constant6/1 -> Switch/3, Switch/1

== system Charge_1_V1_experiment/HANcoder STM32 Target - E407-STM32 algorithm/Current_SP/Subsystem2/Voltage_Control/3phase/Subsystem1/Subsystem ==
  In1 : Inport
  In2 : Inport  Port=2
  In3 : Inport  Port=3
  In4 : Inport  Port=4
  In5 : Inport  Port=5
  In6 : Inport  Port=6
  In7 : Inport  Port=7
  In8 : Inport  Port=8
  Constant10 : Constant  Value=5  OutDataTypeStr=single  SampleTime=-1
  Constant6 : Constant  OutDataTypeStr=single  SampleTime=-1
  Constant7 : Constant  Value=2  OutDataTypeStr=single  SampleTime=-1
  Constant8 : Constant  Value=3  OutDataTypeStr=single  SampleTime=-1
  Constant9 : Constant  Value=4  OutDataTypeStr=single  SampleTime=-1
  Logical Operator : Logic  AllPortsSameDT=off  OutDataTypeStr=boolean
  Logical Operator1 : Logic  AllPortsSameDT=off  OutDataTypeStr=boolean
  Logical Operator2 : Logic  AllPortsSameDT=off  OutDataTypeStr=boolean
  Switch{,1..4} (5 alike) : Switch  Criteria=u2 > Threshold
  Out1 : Outport
  wires:
  Constant6/1 -> Switch/1, Switch/3
  In7/1 -> Logical Operator2/2
  In6/1 -> Logical Operator2/1
  In3/1 -> Logical Operator/2
  In5/1 -> Logical Operator1/2
  In2/1 -> Logical Operator/1
  In4/1 -> Logical Operator1/1
  Logical Operator1/1 -> Switch2/2
  In1/1 -> Switch/2
  Switch1/1 -> Switch2/3
  Constant9/1 -> Switch3/1
  Switch4/1 -> Out1/1
  In8/1 -> Switch4/2
  Logical Operator/1 -> Switch1/2
  Switch/1 -> Switch1/3
  Constant7/1 -> Switch1/1
  Constant10/1 -> Switch4/1
  Constant8/1 -> Switch2/1
  Switch2/1 -> Switch3/3
  Switch3/1 -> Switch4/3
  Logical Operator2/1 -> Switch3/2

== system Charge_1_V1_experiment/HANcoder STM32 Target - E407-STM32 algorithm/Energy Meter/Energy_Meter_Recieve/Subsystem1/Power_Meter/Current_Phase1/Read_Gyro1 ==
  note: 01040000000271CB
  In1 : Inport
  Trigger : TriggerPort  VariantControl=Variant
  UART send : Subsystem  Tag=HANcoder_TARGET_STM32_E407  AncestorBlock=HANcoder_STM32_Target/STM32-E407/UART/UART send  mask(UART send){channel=UART1: CON3 - D1 & D0, useStatusOut=off, tsamp=-1}
      mask prompts: useStatusOut "Use status outport"; tsamp "Sample time"
      mask help:
      | Function
      | ==========
      | Transmits a byte on the UART communication interface.
      |
      | Parameters per channel
      | ======================
      | - Select channel (TX & RX)
      | - Select if the status output should be enabled.
      |
      | Inputs
      | ======
      | - The byte to send
      |
      | Outputs
      | =======
      | - When the status output is 0, the byte could not be transmitted. Probably
      |   because the transmit buffer was configured too small.
      mask init:
      | uartChannelInfoStr = sfcn_uart_send_mcb(2, channel, useStatusOut);
      settings: MoveFcn=drawLogos
      mask Help: web('sfcn_uart_send.html')
      mask TypeOptions channel: UART1: CON3 - D1 & D0 | UART2: CON PD - 8 & 9 | UART3: CON PD - 11 & 12 | UART6: UEXT - 3 & 4
      mask Display: fprintf('UART send\n%s', uartChannelInfoStr);patch([245 251 251],[8 14 2],[1 0 0]);patch([253 253 259],[14 2 8],[0 0 0.35]);
  wires:
  In1/1 -> UART send/1(In1)
